simulink model "BallBeam"  (Simulink 7.5)
settings: Solver=ode45  StartTime=0.0  StopTime=5  MaxStep=1e-4  RelTol=1e-3
InitFcn:
  | g = 9.81; %gravitational constant
  | 
  | % showVR = 1; %show VR world
  | % alpha_init = 0; %initial condition
  | % x_init = 0; %initial condition
libraries: vrlib x1
CloseFcn:
  | vrclose all;
  | clear figureVR worldVR;
settings Model: Creator=H  LastModifiedBy=michal
settings OptimizationCC: InitFltsAndDblsToZero=on
settings DebuggingCC: SaveWithParameterizedLinksMsg=none  SignalResolutionControl=TryResolveAllWithWarning  StrictBusMsg=Warning
settings GRTTargetCC: TargetFcnLib=ansi_tfl_tmw.mat

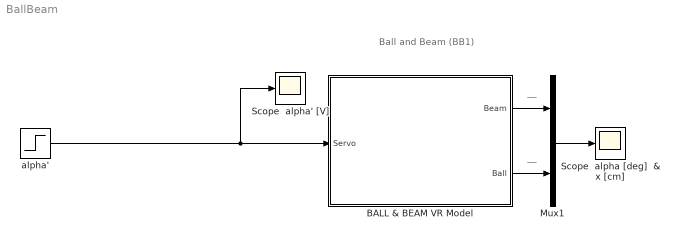
== system BallBeam ==
  note: Ball and Beam (BB1)
  note: __
  note: __
  BALL & BEAM VR Model : Subsystem  mask(Ball and Beam (BB1) in laboratory K26){showVR=on, sfcnParam1=0, sfcnParam2=0}
      mask prompts: showVR "Show VirtualWorld?"; sfcnParam1 "Initial angle of the beam  alpha(0)  [deg]"; sfcnParam2 "Initial position of the ball  x(0) [cm]"
      mask help: Ball and Beam (BB1) in laboratory K26 - Virtual Reality
      mask Help:
      | Ball and Beam in laboratory K26 - Virtual Reality. <br><br>
      | 
      | 
      | This is a virtual model of the Ball and Beam apparatus in Laboratory of automatic control
      | theory&nbsp;26 (<a href="http://support.dce.felk.cvut.cz/lab26/" target="_blank">http://support.dce.felk.cvut.cz/lab26/</a>),
      | which consists of a&nbsp;beam and a&nbsp;ball. The&nbsp;ball is moving on the&nbsp;beam. The&nbsp;beam angle
      | is controlled by the&nbsp;input&nbsp;<em>&alpha;'</em>&nbsp;[V] (setpoint for the&nbsp;angle of the&nbsp;beam -
      | the&nbsp;beam is in closed loop with a&nbsp;P-controller). <br><br>
      | 
      | The system input is the&nbsp;setpoint of the&nbsp;angle of the&nbsp;beam&nbsp;<em>&alpha;'</em>&nbsp; [V].
      | The&nbsp;system outputs are the&nbsp;real beam angle&nbsp;<em>&alpha</em>&nbsp;[deg] and the&nbsp;ball
      | possition&nbsp;<em>x</em>&nbsp;[cm]. More information can be found on the website
      | <a href="http://support.dce.felk.cvut.cz/lab26/" target="_blank">http://support.dce.felk.cvut.cz/lab26/</a>.<br><br>
      | 
      | 
      | In the mask of the model, it can be set:
      | <ul>
      | <li>Initial angle of the beam</li>
      | <li>Initial position of the ball.</li>
      | </ul><br><br>
      | 
      | 
      | Copyright: 2008, Jan Kricka, Jirka Roubal, Petr Husek.
      mask CallbackString:
      | if strcmp('off',get_param(gcb,'showVR'))
      |     vrclose all;
      | else
      |     if exist('figureVR')==0
      |         figureVR = vrfigure;
      |     end
      |     if exist('worldVR')==0
      |         worldVR = vrworld('BallBeam_VR.WRL');
      |     end
      | 	if isvalid(figureVR)==0
      |         open(worldVR);
      |         figureVR = vrfigure(worldVR,[650 80 550 350]);
      | 	end
      | end||
      mask Display:
      | image(imread('BallBeam_Image.jpg'));
      | port_label ('input',1,'alpha'' [V]');
      | port_label ('output',1,'alpha [deg]');
      | port_label ('output',2,'x [cm]');
  Mux1 : Mux  Inputs=2
  Scope  alpha [deg]  & x [cm] : Scope
      settings: TimeRange=5  YMin=-10  YMax=50  SaveName=ty  DataFormat=Array  MaxDataPoints=500000
  Scope  alpha' [V] : Scope
      settings: TimeRange=5  YMin=-10  YMax=10  SaveName=tu  DataFormat=Array  MaxDataPoints=500000
  alpha' : Step  After=5  SampleTime=0
  wires:
  BALL & BEAM VR Model/1(Beam) -> Mux1/1
  Mux1/1 -> Scope  alpha [deg]  & x [cm]/1
  BALL & BEAM VR Model/2(Ball) -> Mux1/2
  alpha'/1 -> Scope  alpha' [V]/1, BALL & BEAM VR Model/1(Servo)

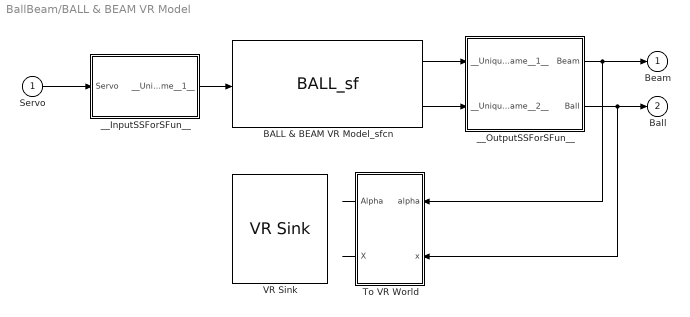
== system BallBeam/BALL & BEAM VR Model ==
  Servo : Inport  OutDataType=sfix(16)  OutScaling=2^0
  BALL & BEAM VR Model_sfcn : S-Function  FunctionName=BALL_sf  Parameters=sfcnParam1, sfcnParam2  SFunctionModules=""  EnableBusSupport=off  mask{rtw_sf_name=BALL_sf, showVar=off, sfcnParam1=sfcnParam1, sfcnParam2=sfcnParam2}
      mask prompts: rtw_sf_name "Generated S-function name (model_sf):"; showVar "Show module list"; sfcnParam1 "alpha_init:"; sfcnParam2 "x_init:"
      mask help: Real-Time Workshop generated S-function.
      mask init:
      | displist = '';
      | if ~strcmp(get_param(gcb, 'FunctionName'), rtw_sf_name);
      |   set_param(gcb, 'FunctionName', rtw_sf_name);
      | end
      | % Check if we are generating RTW code
      | rtw_mode = false;
      | if strcmpi(get_param(bdroot(gcb),'SimulationStatus'),'Initializing')
      | 	rtw_mode = strcmpi(get_param(bdroot(gcb),'BuildingRTWCode'),'on') && ...
      | 		~strcmpi(get_param(bdroot(gcb),'TargetStyle'),'SimulationTarget');
      | end
      | if showVar || rtw_mode
      | 	if exist('rtwsfunc') == 2 | exist('rtwsfunc') == 6
      | 		tmplist = rtwsfunc(rtw_sf_name,gcb);
      | 		tmplist = ['\nList of Modules:\n', tmplist];
      | 	elseif showVar
      | 		tmplist = '\nList of Modules:\nRTW not licensed\n';
      |  	end
      | end
      | if showVar
      |   displist = tmplist;
      | end
      settings: CopyFcn=set_param(gcb,'LinkStatus','none');
      mask Help: helpview([docroot,'\toolbox\rtw\helptargets.map'],'rtw_Sfunc_target');
      mask Display:
      | port_label('input',1,'Servo');
      | port_label('output',1,'Beam');
      | port_label('output',2,'Ball');
  To VR World : Subsystem
  VR Sink : vrlib/VR Sink  InstantiateOnLoad=on  SampleTime=0.1  ViewEnable=on  RemoteChange=off  RemoteView=on  FieldsWritten=Beam.rotation.4.1.double#ball.translation.3.1.double  WorldFileName=BallBeam_VR.WRL  AutoView=off  VideoDimensions=[]
  __InputSSForSFun__ : Subsystem
  __OutputSSForSFun__ : Subsystem
  Beam : Outport  PortDimensions=1  SampleTime=[-1 0]  DataType=double  OutDataType=sfix(16)  OutScaling=2^0  OutDataTypeStr=double
  Ball : Outport  Port=2  PortDimensions=1  SampleTime=[-1 0]  DataType=double  OutDataType=sfix(16)  OutScaling=2^0  OutDataTypeStr=double
  wires:
  To VR World/2(X) -> ?
  To VR World/1(Alpha) -> ?
  __OutputSSForSFun__/2(Ball) -> To VR World/2(x), Ball/1
  __OutputSSForSFun__/1(Beam) -> To VR World/1(alpha), Beam/1
  BALL & BEAM VR Model_sfcn/2 -> __OutputSSForSFun__/2(__UniqueInportName__2__)
  BALL & BEAM VR Model_sfcn/1 -> __OutputSSForSFun__/1(__UniqueInportName__1__)
  __InputSSForSFun__/1(__UniqueOutportName__1__) -> BALL & BEAM VR Model_sfcn/1
  Servo/1 -> __InputSSForSFun__/1(Servo)

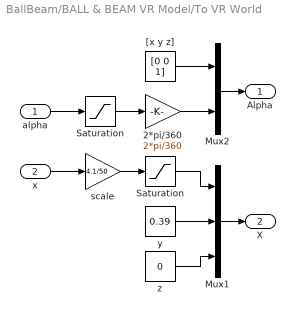
== system BallBeam/BALL & BEAM VR Model/To VR World ==
  alpha : Inport  OutDataType=sfix(16)  OutScaling=2^0
  x : Inport  Port=2  OutDataType=sfix(16)  OutScaling=2^0
  2*pi/360 : Gain  Gain=2*pi/360  ParameterDataType=sfix(16)  ParameterScaling=2^0  OutDataType=sfix(16)  OutScaling=2^0
  Mux1 : Mux  Inputs=3
  Mux2 : Mux  Inputs=2
  Saturation : Saturate  UpperLimit=4.1  LowerLimit=-4.1
  "Saturation " : Saturate  UpperLimit=15  LowerLimit=-15
  "[x y z]" : Constant  Value=[0 0 1]  OutDataType=sfix(16)  OutScaling=2^0
  scale : Gain  Gain=4.1/50  ParameterDataType=sfix(16)  ParameterScaling=2^0  OutDataType=sfix(16)  OutScaling=2^0
  y : Constant  Value=0.39  OutDataType=sfix(16)  OutScaling=2^0
  z : Constant  Value=0  OutDataType=sfix(16)  OutScaling=2^0
  Alpha : Outport  OutDataType=sfix(16)  OutScaling=2^0
  X : Outport  Port=2  OutDataType=sfix(16)  OutScaling=2^0
  wires:
  Mux1/1 -> X/1
  x/1 -> scale/1
  alpha/1 -> "Saturation "/1
  Mux2/1 -> Alpha/1
  scale/1 -> Saturation/1
  y/1 -> Mux1/2
  z/1 -> Mux1/3
  "[x y z]"/1 -> Mux2/1
  Saturation/1 -> Mux1/1
  2*pi/360/1 -> Mux2/2
  "Saturation "/1 -> 2*pi/360/1

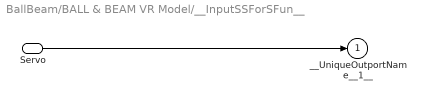
== system BallBeam/BALL & BEAM VR Model/__InputSSForSFun__ ==
  Servo : Inport  OutDataType=sfix(16)  OutScaling=2^0
  __UniqueOutportName__1__ : Outport  OutDataType=sfix(16)  OutScaling=2^0
  wires:
  Servo/1 -> __UniqueOutportName__1__/1

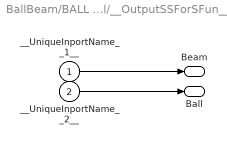
== system BallBeam/BALL & BEAM VR Model/__OutputSSForSFun__ ==
  __UniqueInportName__1__ : Inport  OutDataType=sfix(16)  OutScaling=2^0
  __UniqueInportName__2__ : Inport  Port=2  OutDataType=sfix(16)  OutScaling=2^0
  Beam : Outport  PortDimensions=1  SampleTime=[-1 0]  DataType=double  OutDataType=sfix(16)  OutScaling=2^0  OutDataTypeStr=double
  Ball : Outport  Port=2  PortDimensions=1  SampleTime=[-1 0]  DataType=double  OutDataType=sfix(16)  OutScaling=2^0  OutDataTypeStr=double
  wires:
  __UniqueInportName__2__/1 -> Ball/1
  __UniqueInportName__1__/1 -> Beam/1
